simulink model "tricycle"  (R2021a)
settings: Solver=VariableStepAuto  StartTime=0.0  StopTime=10.0  RelTol=1e-3
settings Model: Creator=francesco  LastModifiedBy=francesco

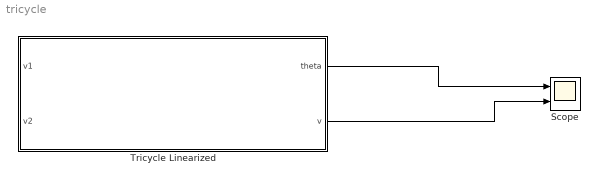
== system tricycle ==
  Scope : Scope  NumInputPorts=2
  Tricycle Linearized : Subsystem
  wires:
  Tricycle Linearized/1(theta) -> Scope/1
  Tricycle Linearized/2(v) -> Scope/2

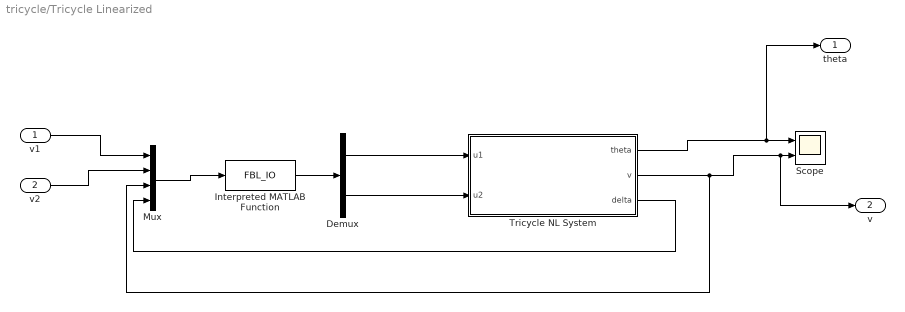
== system tricycle/Tricycle Linearized ==
  v1 : Inport
  v2 : Inport  Port=2
  Demux : Demux  Outputs=2
  Interpreted MATLAB Function : MATLABFcn  MATLABFcn=FBL_IO  OutputDimensions=2
  Mux : Mux
  Scope : Scope  NumInputPorts=2
  Tricycle NL System : Subsystem
  theta : Outport
  v : Outport  Port=2
  wires:
  Mux/1 -> Interpreted MATLAB Function/1
  v2/1 -> Mux/2
  v1/1 -> Mux/1
  Demux/1 -> Tricycle NL System/1(u1)
  Tricycle NL System/1(theta) -> theta/1, Scope/1
  Tricycle NL System/2(v) -> Mux/3, v/1, Scope/2
  Interpreted MATLAB Function/1 -> Demux/1
  Demux/2 -> Tricycle NL System/2(u2)
  Tricycle NL System/3(delta) -> Mux/4

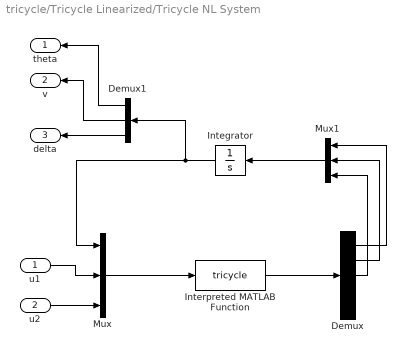
== system tricycle/Tricycle Linearized/Tricycle NL System ==
  u1 : Inport
  u2 : Inport  Port=2
  Demux : Demux  Outputs=5
  Demux1 : Demux  Outputs=3
  Integrator : Integrator  InitialCondition=[0 0 0]
  Interpreted MATLAB Function : MATLABFcn  MATLABFcn=tricycle  OutputDimensions=5
  Mux : Mux  Inputs=3
  Mux1 : Mux  Inputs=3
  theta : Outport
  v : Outport  Port=2
  delta : Outport  Port=3
  wires:
  Mux1/1 -> Integrator/1
  Demux/1 -> Mux1/1
  Demux1/1 -> theta/1
  Interpreted MATLAB Function/1 -> Demux/1
  Integrator/1 -> Mux/1, Demux1/1
  Mux/1 -> Interpreted MATLAB Function/1
  Demux/2 -> Mux1/2
  Demux/3 -> Mux1/3
  Demux1/2 -> v/1
  u1/1 -> Mux/2
  u2/1 -> Mux/3
  Demux1/3 -> delta/1
